simulink model "Fake_Algorithm_Control_1"  (Simulink 7.5)
settings: Solver=ode45  StartTime=0.0  StopTime=10.0  RelTol=1e-3
undefined symbols (not defined in the file or in its folder): ctrller
settings Model: Creator=sriddle  LastModifiedBy=sriddle

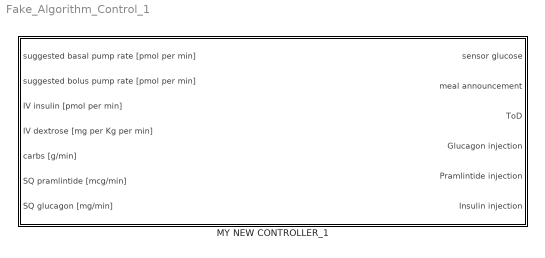
== system Fake_Algorithm_Control_1 ==
  MY NEW CONTROLLER_1 : Subsystem

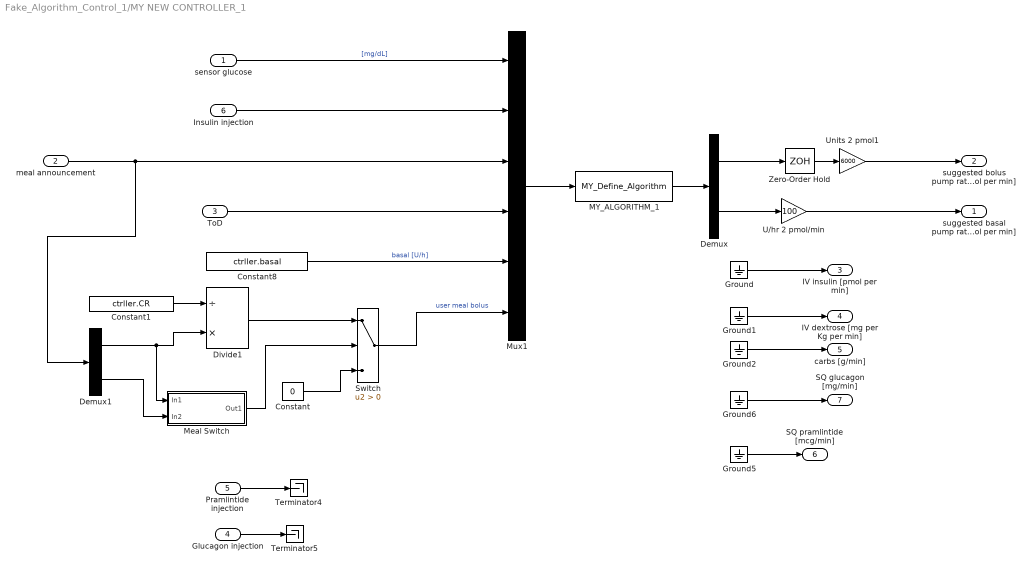
== system Fake_Algorithm_Control_1/MY NEW CONTROLLER_1 ==
  sensor glucose : Inport  OutDataType=sfix(16)  OutScaling=2^0
  meal announcement : Inport  Port=2  OutDataType=sfix(16)  OutScaling=2^0
  ToD : Inport  Port=3  OutDataType=sfix(16)  OutScaling=2^0
  Glucagon injection : Inport  Port=4
  Pramlintide injection : Inport  Port=5
  Insulin injection : Inport  Port=6  OutDataType=sfix(16)  OutScaling=2^0
  Constant : Constant  Value=0  OutDataType=sfix(16)  OutScaling=2^0
  Constant1 : Constant  Value=ctrller.CR  OutDataType=sfix(16)  OutScaling=2^0
  Constant8 : Constant  Value=ctrller.basal  OutDataType=sfix(16)  OutScaling=2^0
  Demux : Demux  Outputs=2
  Demux1 : Demux  Outputs=2
  Divide1 : Product  Inputs=/*  OutDataType=sfix(16)  OutScaling=2^-10
  Ground{,1..2,5..6} (5 alike) : Ground
  MY_ALGORITHM_1 : MATLABFcn  InitFcn=clear global  MATLABFcn=MY_Define_Algorithm  OutputDimensions=2
  Meal Switch : Subsystem
  Mux1 : Mux  Inputs=6
  Switch : Switch  Criteria=u2 > Threshold  OutDataType=sfix(16)  OutScaling=2^0
  Terminator4 : Terminator
  Terminator5 : Terminator
  U/hr 2 pmol/min : Gain  Gain=100  ParameterDataType=sfix(16)  ParameterScaling=2^0  OutDataType=sfix(16)  OutScaling=2^0
  Units 2 pmol1 : Gain  Gain=6000  ParameterDataType=sfix(16)  ParameterScaling=2^0  OutDataType=sfix(16)  OutScaling=2^0
  Zero-Order Hold : ZeroOrderHold  SampleTime=-1
  suggested basal pump rate [pmol per min] : Outport  OutDataType=sfix(16)  OutScaling=2^0
  suggested bolus pump rate [pmol per min] : Outport  Port=2  OutDataType=sfix(16)  OutScaling=2^0
  IV insulin [pmol per min] : Outport  Port=3  OutDataType=sfix(16)  OutScaling=2^0
  IV dextrose [mg per Kg per min] : Outport  Port=4  OutDataType=sfix(16)  OutScaling=2^0
  carbs [g/min] : Outport  Port=5  OutDataType=sfix(16)  OutScaling=2^0
  SQ pramlintide [mcg/min] : Outport  Port=6
  SQ glucagon [mg/min] : Outport  Port=7
  wires:
  MY_ALGORITHM_1/1 -> Demux/1
  Mux1/1 -> MY_ALGORITHM_1/1
  Demux/1 -> Zero-Order Hold/1
  Demux/2 -> U/hr 2 pmol/min/1
  ToD/1 -> Mux1/4
  sensor glucose/1 -> Mux1/1  "[mg/dL]"
  Insulin injection/1 -> Mux1/2
  Constant8/1 -> Mux1/5  "basal [U/h]"
  Zero-Order Hold/1 -> Units 2 pmol1/1
  Constant1/1 -> Divide1/1
  Demux1/1 -> Divide1/2, Meal Switch/1(In1)
  Demux1/2 -> Meal Switch/2(In2)
  Meal Switch/1(Out1) -> Switch/2
  Constant/1 -> Switch/3
  Divide1/1 -> Switch/1
  Switch/1 -> Mux1/6  "user meal bolus"
  U/hr 2 pmol/min/1 -> suggested basal pump rate [pmol per min]/1
  meal announcement/1 -> Mux1/3, Demux1/1
  Ground2/1 -> carbs [g/min]/1
  Ground1/1 -> IV dextrose [mg per Kg per min]/1
  Ground/1 -> IV insulin [pmol per min]/1
  Units 2 pmol1/1 -> suggested bolus pump rate [pmol per min]/1
  Ground6/1 -> SQ glucagon [mg/min]/1
  Ground5/1 -> SQ pramlintide [mcg/min]/1
  Pramlintide injection/1 -> Terminator4/1
  Glucagon injection/1 -> Terminator5/1

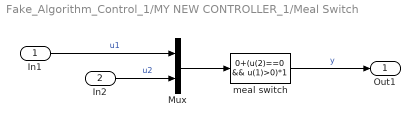
== system Fake_Algorithm_Control_1/MY NEW CONTROLLER_1/Meal Switch ==
  In1 : Inport
  In2 : Inport  Port=2
  Mux : Mux  Inputs=2
  meal switch : MATLABFcn  MATLABFcn=0+(u(2)==0 && u(1)>0)*1
  Out1 : Outport
  wires:
  Mux/1 -> meal switch/1
  In1/1 -> Mux/1  "u1"
  meal switch/1 -> Out1/1  "y"
  In2/1 -> Mux/2  "u2"
